simulink model "character_encoder"  (R2021a)
settings: Solver=VariableStepAuto  StartTime=0.0  StopTime=(N-1)/Fs  RelTol=1e-3
values from neighbouring files (symbols this model uses):
  fCase = 100    [Script.m]
  fHigh = frequencies(row, 3)    [Script.m]
  fLow = frequencies(row, 1)    [Script.m]
  fMid = frequencies(row, 2)    [Script.m]
  Fs = 8000    [Script.m]    (also in character_signals.mat)
settings Model: Creator=amirm  LastModifiedBy=amirm

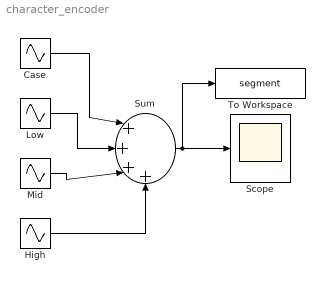
== system character_encoder ==
  Case : Sin  Amplitude=0.25  Frequency=2*pi*fCase  Phase=pi/2  SampleTime=1/Fs
  High : Sin  Amplitude=0.25  Frequency=2*pi*fHigh  Phase=pi/2  SampleTime=1/Fs
  Low : Sin  Amplitude=0.25  Frequency=2*pi*fLow  Phase=pi/2  SampleTime=1/Fs
  Mid : Sin  Amplitude=0.25  Frequency=2*pi*fMid  Phase=pi/2  SampleTime=1/Fs
  Scope : Scope
  Sum : Sum  Inputs=|++++
  To Workspace : ToWorkspace  VariableName=segment  SampleTime=-1
  wires:
  Case/1 -> Sum/1
  Low/1 -> Sum/2
  Mid/1 -> Sum/3
  High/1 -> Sum/4
  Sum/1 -> To Workspace/1, Scope/1
